simulink model "ds1_plant"  (R2019a)
settings: Solver=ode14x  StartTime=0  StopTime=0.166  FixedStep=.00001  RelTol=1e-3  EnableMultiTasking=on
model workspace (MAT data in the model file):
  Ankle_L_D = 0.125126243033
  Ankle_L_S = 0.0328154604487
  Ankle_R_D = 0.245807097642
  Ankle_R_S = 0.0328154604487
  BeginTimePlantModel = 0.1577
  F_C = 0.0618
  F_H = 0.107
  F_I = 0.0129
  F_L = 0.2471
  F_M = 1.2499
  F_W = 0.11
  GRF_HD = 941.037069119
  GRF_HS = 1691.11560066
  GRF_VD = 12300.8672242
  GRF_VS = 76710.3574634
  HAT_I = 4.3688
  HAT_L = 0.549
  HAT_M = 58.9152
  HAT_a = 0.2
  HAT_b = 0.13
  Hip_L_D = 0.0332143791481
  Hip_L_S = 0.0516603438036
  Hip_R_D = 0.145088103411
  Hip_R_S = 0.15911410017
  Knee_L_D = 0.0558982452805
  Knee_L_S = 0.00250387295429
  Knee_R_D = 0.0619293882143
  Knee_R_S = 0.0623339259595
  M : struct (value not decoded)
  S_I = 0.073
  S_L = 0.447
  S_M = 4.0083
  S_R1 = 0.06
  S_R2 = 0.08
  T_I = 0.2042
  T_L = 0.476
  T_M = 8.6199999
  T_R1 = 0.08
  T_R2 = 0.1
  bodymass = 2.85423037717
  p_stance_ankle = 14.9539905036
  p_stance_hip = -24.9413676415
  p_stance_knee = -2.50807459996
  p_swing_ankle = 4.11757124464
  p_swing_hip = 18.3000604838
  p_swing_knee = -3.41741510381
  polyfit_stance_ankle = [-863347.977095 222377.922877 -7468.35453889 -9.40558010807 -153.06789694]
  polyfit_stance_hip = [-279786636.688 114363391.625 -15725654.0525 856134.662579 -22930.0516399 481.110496147 63.2694363354]
  polyfit_stance_knee = [-122862314.114 52903969.6705 -7988612.27678 487806.049871 -8969.32141641 330.337585729 -54.0526736443]
  polyfit_swing_ankle = [49510154320.8 -30205907167.6 7312588550.85 -888915044.437 56385922.5861 -1769074.37171 25613.4020917 -113.306543933 -1.03720591697]
  polyfit_swing_hip = [538683495113 -366532634246 101719653645 -14750073882.9 1184454520.37 -50949861.1242 1019832.60417 -6310.84925925 -38.0907282261]
  polyfit_swing_knee = [352478408737 -233011269241 62650744932.5 -8775138187.04 678489689.503 -28060179.8998 545151.783137 -3282.03325692 -26.455631467]
  stance_hip_D = -0.1
  stance_hip_I = 0
  stance_hip_P = -1
  swing_hip_D = -0.1
  swing_hip_I = 0
  swing_hip_P = -1
  u_stance_ankle = [-114.620040933 -149.993105962 -149.909908907 -149.999889888 -149.999957965 -149.999973006]
  u_stance_knee = [-4.39803453247 -27.0219790006 -26.9634089217 -27.1316089475 -27.1524298795 -13.1129133696]
  u_swing_ankle = [7.00267747461 -1.55234842214 7.02970023555 7.00586724227 7.06043061801 0.00199706532211]
  u_swing_knee = [-10.6470024823 -8.89238612545 -13.3071794193 -13.064145722 -14.1272814659 -14.0994649135]
  w_stance_ankle = -19.9817779
  w_stance_hip = 18.2437977096
  w_stance_knee = 116.890654217
  w_swing_ankle = -56.5478745686
  w_swing_hip = 29.8978013919
  w_swing_knee = 6.91676966665
  x_planar_p = 0
  x_planar_v = 0
  y_planar_p = 0
  y_planar_v = 0
  yout = [8.16988597066 8.1627557225 8.15559878707 8.14841513681 8.14120474348 8.13396757813 8.12670361115 8.11941281227 8.1120951506 8.10475059463 8.09737911226 8.08998067083 ... (8000 elements, 1000x8)]
  z_planar_p = -10.3139246991
  z_planar_w = -47.4942945829
symbols that are objects in the model workspace (value not decoded): M
undefined symbols (not defined in the file or in its folder): X, Y, Z
libraries: nesl_utility x88, sm_lib x51, fl_lib x24, fl_ps_legacy_lib x16, simulink x4
(part 3 of 4)

== system ds1_plant/lead shank ==
  Rigid  Transform : sm_lib/Frames and Transforms/Rigid Transform  TranslationMethod=None  TranslationStandardOffset=S_L  TranslationLengthUnit=m  TranslationStandardAxis=+Z  TranslationCartesianOffset=[0 0 0]  TranslationROffset=0  TranslationROffsetUnits=m  TranslationZOffset=0  TranslationZOffsetUnits=m  TranslationThetaOffset=0  TranslationThetaOffsetUnits=deg  RotationMethod=StandardAxis  RotationAngleUnits=deg  RotationStandardAxis=+Y  RotationAngle=90  RotationArbitraryAxis=[0 0 1]  FollAlignAxisA=+X  BaseAlignAxisA=+Y  FollAlignAxisB=+Y  BaseAlignAxisB=+Z  RotationSequenceAxes=FollowerAxes  RotationSequence=XYX  RotationSequenceAngles=[0 0 0]  RotationSequenceAnglesUnits=deg  RotationMatrix=[1 0 0; 0 1 0; 0 0 1]
  Rigid  Transform1 : sm_lib/Frames and Transforms/Rigid Transform  TranslationMethod=StandardAxis  TranslationStandardOffset=S_L  TranslationLengthUnit=m  TranslationStandardAxis=+Z  TranslationCartesianOffset=[0 0 0]  TranslationROffset=0  TranslationROffsetUnits=m  TranslationZOffset=0  TranslationZOffsetUnits=m  TranslationThetaOffset=0  TranslationThetaOffsetUnits=deg  RotationMethod=StandardAxis  RotationAngleUnits=deg  RotationStandardAxis=+Y  RotationAngle=90  RotationArbitraryAxis=[0 0 1]  FollAlignAxisA=+X  BaseAlignAxisA=+Y  FollAlignAxisB=+Y  BaseAlignAxisB=+Z  RotationSequenceAxes=FollowerAxes  RotationSequence=XYX  RotationSequenceAngles=[0 0 0]  RotationSequenceAnglesUnits=deg  RotationMatrix=[1 0 0; 0 1 0; 0 0 1]
  Solid : sm_lib/Body Elements/Solid  InertiaType=Custom  Mass=S_M  MassUnits=kg  CenterOfMass=[0 0 0.567*S_L]  CenterOfMassUnits=m  MomentsOfInertia=[S_I .001 .001]  MomentsOfInertiaUnits=kg*m^2  ProductsOfInertia=[0 0 0]  ProductsOfInertiaUnits=kg*m^2  BasedOnType=Density  Density=0  DensityUnits=kg/(m^3)  DoExposeReferenceFrame=on  SerializedFrames=<Frames/>  GraphicType=FromGeometry  MarkerShape=Sphere  MarkerSize=10  MarkerSizeUnits=m  GraphicVisPropType=SimpleVisualProperties  GraphicDiffuseColor=[0.0 0.4 1.0]  GraphicSpecularColor=[0.5 0.5 0.5 1.0]  GraphicAmbientColor=[0.15 0.15 0.15 1.0]  GraphicEmissiveColor=[0.0 0.0 0.0 1.0]  GraphicShininess=75  GraphicOpacity=1.0  GeometryShape=GeneralSolidOfRevolution  RectangleSize=[1 1]  RectangleSizeUnits=m  BrickDimensions=[1 1 1]  BrickDimensionUnits=m  CylinderRadius=1  CylinderRadiusUnits=m  CylinderLength=1  CylinderLengthUnits=m  SphereRadius=1  SphereRadiusUnits=m  EllipsoidRadii=[1 1 1]  EllipsoidRadiiUnits=m  ExtrusionCrossSection=[1 1; -1 1; -1 -1; 1 -1]  ExtrusionCrossSectionUnits=m  ExtrusionLength=1  ExtrusionLengthUnits=m  PolygonNumSides=3  PolygonOuterRadius=1  PolygonOuterRadiusUnits=m  ExtGeomFileType=STEP  ExtGeomFileUnits=m  RevolutionCrossSection=S_cross_section  RevolutionCrossSectionUnits=m  RevolutionExtent=Full  RevolutionAngle=180  RevolutionAngleUnits=deg
  B : PMIOPort  Side=Right
  F : PMIOPort  Port=2  Side=Left
  connections:
  B/RConn1 -- Rigid  Transform/RConn1
  Rigid  Transform/LConn1 -- Rigid  Transform1/LConn1 -- Solid/RConn1
  F/RConn1 -- Rigid  Transform1/RConn1

== system ds1_plant/lead thigh ==
  Rigid  Transform : sm_lib/Frames and Transforms/Rigid Transform  TranslationMethod=None  TranslationStandardOffset=T_L  TranslationLengthUnit=m  TranslationStandardAxis=+Z  TranslationCartesianOffset=[0 0 0]  TranslationROffset=0  TranslationROffsetUnits=m  TranslationZOffset=0  TranslationZOffsetUnits=m  TranslationThetaOffset=0  TranslationThetaOffsetUnits=deg  RotationMethod=StandardAxis  RotationAngleUnits=deg  RotationStandardAxis=+Y  RotationAngle=90  RotationArbitraryAxis=[0 0 1]  FollAlignAxisA=+X  BaseAlignAxisA=+Y  FollAlignAxisB=+Y  BaseAlignAxisB=+Z  RotationSequenceAxes=FollowerAxes  RotationSequence=XYX  RotationSequenceAngles=[0 0 0]  RotationSequenceAnglesUnits=deg  RotationMatrix=[1 0 0; 0 1 0; 0 0 1]
  Rigid  Transform1 : sm_lib/Frames and Transforms/Rigid Transform  TranslationMethod=StandardAxis  TranslationStandardOffset=T_L  TranslationLengthUnit=m  TranslationStandardAxis=+Z  TranslationCartesianOffset=[0 0 0]  TranslationROffset=0  TranslationROffsetUnits=m  TranslationZOffset=0  TranslationZOffsetUnits=m  TranslationThetaOffset=0  TranslationThetaOffsetUnits=deg  RotationMethod=StandardAxis  RotationAngleUnits=deg  RotationStandardAxis=+Y  RotationAngle=90  RotationArbitraryAxis=[0 0 1]  FollAlignAxisA=+X  BaseAlignAxisA=+Y  FollAlignAxisB=+Y  BaseAlignAxisB=+Z  RotationSequenceAxes=FollowerAxes  RotationSequence=XYX  RotationSequenceAngles=[0 0 0]  RotationSequenceAnglesUnits=deg  RotationMatrix=[1 0 0; 0 1 0; 0 0 1]
  Thigh : sm_lib/Body Elements/Solid  InertiaType=Custom  Mass=T_M  MassUnits=kg  CenterOfMass=[0 0 0.567*T_L]  CenterOfMassUnits=m  MomentsOfInertia=[T_I .001 .001]  MomentsOfInertiaUnits=kg*m^2  ProductsOfInertia=[0 0 0]  ProductsOfInertiaUnits=kg*m^2  BasedOnType=Density  Density=0  DensityUnits=kg/(m^3)  DoExposeReferenceFrame=on  SerializedFrames=<Frames/>  GraphicType=FromGeometry  MarkerShape=Sphere  MarkerSize=10  MarkerSizeUnits=m  GraphicVisPropType=SimpleVisualProperties  GraphicDiffuseColor=[0.0 0.4 1.0]  GraphicSpecularColor=[0.5 0.5 0.5 1.0]  GraphicAmbientColor=[0.15 0.15 0.15 1.0]  GraphicEmissiveColor=[0.0 0.0 0.0 1.0]  GraphicShininess=75  GraphicOpacity=1.0  GeometryShape=GeneralSolidOfRevolution  RectangleSize=[1 1]  RectangleSizeUnits=m  BrickDimensions=[1 1 1]  BrickDimensionUnits=m  CylinderRadius=[1 2]  CylinderRadiusUnits=m  CylinderLength=1  CylinderLengthUnits=m  SphereRadius=1  SphereRadiusUnits=m  EllipsoidRadii=[1 1 1]  EllipsoidRadiiUnits=m  ExtrusionCrossSection=T_cross_section  ExtrusionCrossSectionUnits=cm  ExtrusionLength=T_L  ExtrusionLengthUnits=cm  PolygonNumSides=3  PolygonOuterRadius=1  PolygonOuterRadiusUnits=m  ExtGeomFileType=STEP  ExtGeomFileUnits=m  RevolutionCrossSection=T_cross_section  RevolutionCrossSectionUnits=m  RevolutionExtent=Full  RevolutionAngle=180  RevolutionAngleUnits=deg
  B : PMIOPort  Side=Right
  F : PMIOPort  Port=2  Side=Left
  connections:
  B/RConn1 -- Rigid  Transform/RConn1
  Rigid  Transform/LConn1 -- Rigid  Transform1/LConn1 -- Thigh/RConn1
  Rigid  Transform1/RConn1 -- F/RConn1

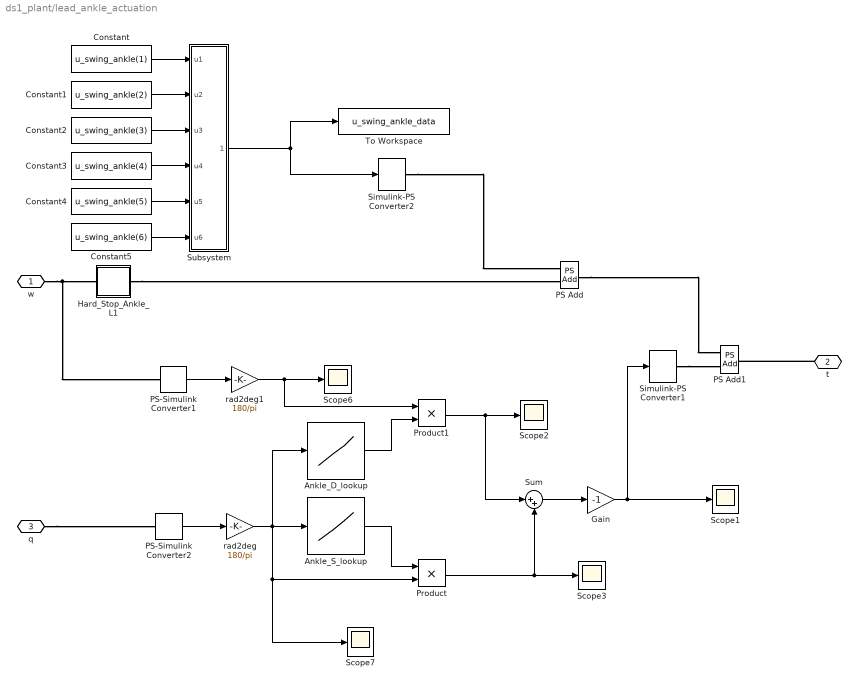
== system ds1_plant/lead_ankle_actuation ==
  Ankle_D_lookup : Lookup_n-D  NumberOfTableDimensions=1  BreakpointsForDimension1=[-45:.01:20]  Table=[exp(linspace(log(1000),log(.01),1000)), zeros(1,4500),exp(linspace(log(.01),log(1000),1001))]  RndMeth=Simplest  InputSameDT=on
  Ankle_S_lookup : Lookup_n-D  NumberOfTableDimensions=1  BreakpointsForDimension1=[-45:.01:20]  Table=[exp(linspace(log(10000),log(.01),1000)), zeros(1,4500),exp(linspace(log(.01),log(10000),1001))]  RndMeth=Simplest  InputSameDT=on
  Constant : Constant  Value=u_swing_ankle(1)
  Constant1 : Constant  Value=u_swing_ankle(2)
  Constant2 : Constant  Value=u_swing_ankle(3)
  Constant3 : Constant  Value=u_swing_ankle(4)
  Constant4 : Constant  Value=u_swing_ankle(5)
  Constant5 : Constant  Value=u_swing_ankle(6)
  Gain : Gain  Gain=-1
  Hard_Stop_Ankle_L1 : Subsystem  mask{upper_bound=((20-p_swing_ankle)*pi)/180, lower_bound=((-45-p_swing_ankle)*pi)/180, contact_stiffness=1e8, contact_damping=5000, initial_angular_position=0}
      mask prompts: upper_bound "Upper Bound"; lower_bound "Lower Bound"; contact_stiffness "Contact Stiffness"; contact_damping "Contact Damping"; initial_angular_position "Initial Angular Position"
  PS Add : fl_ps_legacy_lib/Legacy Physical Signals/Functions/PS Add
      settings: SourceProductName=Simscape  SourceProductBaseCode=SS
  PS Add1 : fl_ps_legacy_lib/Legacy Physical Signals/Functions/PS Add
      settings: SourceProductName=Simscape  SourceProductBaseCode=SS
  PS-Simulink Converter1 : nesl_utility/PS-Simulink Converter  PhysicalDomain=network_engine_domain  SubClassName=ps_output  LeftPortType=input  RightPortType=output  PseudoPeriodic=off  Frequencies=[]  Unit=1  AffineConversion=off
  PS-Simulink Converter2 : nesl_utility/PS-Simulink Converter  PhysicalDomain=network_engine_domain  SubClassName=ps_output  LeftPortType=input  RightPortType=output  PseudoPeriodic=off  Frequencies=[]  Unit=1  AffineConversion=off
  Product : Product  RndMeth=Zero
  Product1 : Product  RndMeth=Zero
  Scope{1..3,6..7} (5 alike) : Scope
  Simulink-PS Converter1 : nesl_utility/Simulink-PS Converter  PhysicalDomain=network_engine_domain  SubClassName=ps_input  LeftPortType=input  RightPortType=output  PseudoPeriodic=off  Frequencies=[]  NoiseDistribution=none  NoiseParameters=[]  Unit=1  AffineConversion=off  FilteringAndDerivatives=zero  SimscapeFilterOrder=1  InputFilterTimeConstant=.001  UdotUserProvided=[]
  Simulink-PS Converter2 : nesl_utility/Simulink-PS Converter  PhysicalDomain=network_engine_domain  SubClassName=ps_input  LeftPortType=input  RightPortType=output  PseudoPeriodic=off  Frequencies=[]  NoiseDistribution=none  NoiseParameters=[]  Unit=1  AffineConversion=off  FilteringAndDerivatives=zero  SimscapeFilterOrder=1  InputFilterTimeConstant=.001  UdotUserProvided=[]
  Subsystem : Subsystem
  Sum : Sum  Inputs=|++
  To Workspace : ToWorkspace  VariableName=u_swing_ankle_data  SampleTime=-1
  rad2deg : Gain  Gain=180/pi
  "rad2deg1 " : Gain  Gain=180/pi
  w : PMIOPort  Side=Right
  t : PMIOPort  Port=2  Side=Left
  q : PMIOPort  Port=3  Side=Right
  wires:
  PS-Simulink Converter1/1 -> "rad2deg1 "/1
  PS-Simulink Converter2/1 -> rad2deg/1
  rad2deg/1 -> Ankle_D_lookup/1, Scope7/1, Product/2, Ankle_S_lookup/1
  Ankle_S_lookup/1 -> Product/1
  "rad2deg1 "/1 -> Product1/1, Scope6/1
  Product1/1 -> Sum/1, Scope2/1
  Product/1 -> Scope3/1, Sum/2
  Sum/1 -> Gain/1
  Gain/1 -> Simulink-PS Converter1/1, Scope1/1
  Ankle_D_lookup/1 -> Product1/2
  Constant/1 -> Subsystem/1(u1)
  Constant1/1 -> Subsystem/2(u2)
  Constant2/1 -> Subsystem/3(u3)
  Constant3/1 -> Subsystem/4(u4)
  Constant4/1 -> Subsystem/5(u5)
  Subsystem/1(Out1) -> To Workspace/1, Simulink-PS Converter2/1
  Constant5/1 -> Subsystem/6(u6)
  connections:
  w/RConn1 -- PS-Simulink Converter1/LConn1 -- Hard_Stop_Ankle_L1/LConn1
  Hard_Stop_Ankle_L1/RConn1 -- PS Add/LConn2
  t/RConn1 -- PS Add1/RConn1
  q/RConn1 -- PS-Simulink Converter2/LConn1
  PS Add/RConn1 -- PS Add1/LConn1
  Simulink-PS Converter1/RConn1 -- PS Add1/LConn2
  Simulink-PS Converter2/RConn1 -- PS Add/LConn1

== system ds1_plant/lead_hip_actuation ==
  HAT_feedback : Inport
  HAT_reference : Constant  Value=0
  Hip_R_Actuation1 : Subsystem
  Scope : Scope
  Sum : Sum  Inputs=|+-
  Swing_hip_PID : Subsystem
  q : PMIOPort  Side=Right
  t : PMIOPort  Port=2  Side=Left
  w : PMIOPort  Port=3  Side=Right
  wires:
  HAT_feedback/1 -> Sum/2
  Sum/1 -> Swing_hip_PID/1(Error)
  HAT_reference/1 -> Sum/1
  Swing_hip_PID/1(Swing_hip_control_moment) -> Scope/1, Hip_R_Actuation1/1(Swing_hip_moment)
  connections:
  q/RConn1 -- Hip_R_Actuation1/RConn2
  t/RConn1 -- Hip_R_Actuation1/LConn1
  w/RConn1 -- Hip_R_Actuation1/RConn1

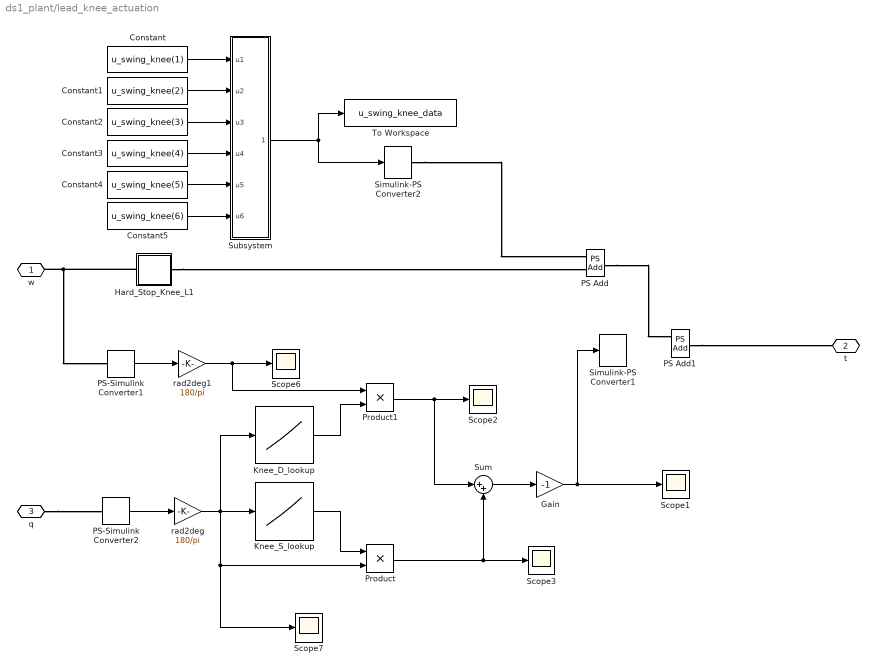
== system ds1_plant/lead_knee_actuation ==
  Constant : Constant  Value=u_swing_knee(1)
  Constant1 : Constant  Value=u_swing_knee(2)
  Constant2 : Constant  Value=u_swing_knee(3)
  Constant3 : Constant  Value=u_swing_knee(4)
  Constant4 : Constant  Value=u_swing_knee(5)
  Constant5 : Constant  Value=u_swing_knee(6)
  Gain : Gain  Gain=-1
  Hard_Stop_Knee_L1 : Subsystem  mask{upper_bound=(-p_swing_knee*pi)/180, lower_bound=((-140-p_swing_knee)*pi)/180, contact_stiffness=1e8, contact_damping=5000, initial_angular_position=0}
      mask prompts: upper_bound "Upper Bound"; lower_bound "Lower Bound"; contact_stiffness "Contact Stiffness"; contact_damping "Contact Damping"; initial_angular_position "Initial Angular Position"
  Knee_D_lookup : Lookup_n-D  NumberOfTableDimensions=1  BreakpointsForDimension1=[-140:.01:0]  Table=[exp(linspace(log(1000),log(.01),1000)), zeros(1,12000),exp(linspace(log(.01),log(1000),1001))]  RndMeth=Simplest  InputSameDT=on
  Knee_S_lookup : Lookup_n-D  NumberOfTableDimensions=1  BreakpointsForDimension1=[-140:.01:0]  Table=[exp(linspace(log(10000),log(.01),1000)), zeros(1,12000),exp(linspace(log(.01),log(10000),1001))]  RndMeth=Simplest  InputSameDT=on
  PS Add : fl_ps_legacy_lib/Legacy Physical Signals/Functions/PS Add
      settings: SourceProductName=Simscape  SourceProductBaseCode=SS
  PS Add1 : fl_ps_legacy_lib/Legacy Physical Signals/Functions/PS Add
      settings: SourceProductName=Simscape  SourceProductBaseCode=SS
  PS-Simulink Converter1 : nesl_utility/PS-Simulink Converter  PhysicalDomain=network_engine_domain  SubClassName=ps_output  LeftPortType=input  RightPortType=output  PseudoPeriodic=off  Frequencies=[]  Unit=1  AffineConversion=off
  PS-Simulink Converter2 : nesl_utility/PS-Simulink Converter  PhysicalDomain=network_engine_domain  SubClassName=ps_output  LeftPortType=input  RightPortType=output  PseudoPeriodic=off  Frequencies=[]  Unit=1  AffineConversion=off
  Product : Product  RndMeth=Zero
  Product1 : Product  RndMeth=Zero
  Scope{1..3,6..7} (5 alike) : Scope
  Simulink-PS Converter1 : nesl_utility/Simulink-PS Converter  PhysicalDomain=network_engine_domain  SubClassName=ps_input  LeftPortType=input  RightPortType=output  PseudoPeriodic=off  Frequencies=[]  NoiseDistribution=none  NoiseParameters=[]  Unit=1  AffineConversion=off  FilteringAndDerivatives=zero  SimscapeFilterOrder=1  InputFilterTimeConstant=.001  UdotUserProvided=[]
  Simulink-PS Converter2 : nesl_utility/Simulink-PS Converter  PhysicalDomain=network_engine_domain  SubClassName=ps_input  LeftPortType=input  RightPortType=output  PseudoPeriodic=off  Frequencies=[]  NoiseDistribution=none  NoiseParameters=[]  Unit=1  AffineConversion=off  FilteringAndDerivatives=zero  SimscapeFilterOrder=1  InputFilterTimeConstant=.001  UdotUserProvided=[]
  Subsystem : Subsystem
  Sum : Sum  Inputs=|++
  To Workspace : ToWorkspace  VariableName=u_swing_knee_data  SampleTime=-1
  rad2deg : Gain  Gain=180/pi
  "rad2deg1 " : Gain  Gain=180/pi
  w : PMIOPort  Side=Right
  t : PMIOPort  Port=2  Side=Left
  q : PMIOPort  Port=3  Side=Right
  wires:
  PS-Simulink Converter1/1 -> "rad2deg1 "/1
  PS-Simulink Converter2/1 -> rad2deg/1
  rad2deg/1 -> Knee_S_lookup/1, Knee_D_lookup/1, Scope7/1, Product/2
  Knee_S_lookup/1 -> Product/1
  "rad2deg1 "/1 -> Product1/1, Scope6/1
  Product1/1 -> Sum/1, Scope2/1
  Product/1 -> Scope3/1, Sum/2
  Sum/1 -> Gain/1
  Gain/1 -> Simulink-PS Converter1/1, Scope1/1
  Knee_D_lookup/1 -> Product1/2
  Constant/1 -> Subsystem/1(u1)
  Constant1/1 -> Subsystem/2(u2)
  Constant2/1 -> Subsystem/3(u3)
  Constant3/1 -> Subsystem/4(u4)
  Constant4/1 -> Subsystem/5(u5)
  Subsystem/1(Out1) -> Simulink-PS Converter2/1, To Workspace/1
  Constant5/1 -> Subsystem/6(u6)
  connections:
  Hard_Stop_Knee_L1/LConn1 -- PS-Simulink Converter1/LConn1 -- w/RConn1
  q/RConn1 -- PS-Simulink Converter2/LConn1
  PS Add/RConn1 -- PS Add1/LConn1
  PS Add1/RConn1 -- t/RConn1
  Hard_Stop_Knee_L1/RConn1 -- PS Add/LConn2
  Simulink-PS Converter2/RConn1 -- PS Add/LConn1

== system ds1_plant/HAT/vCOMCal1 ==
  PS-S : nesl_utility/PS-Simulink Converter  PhysicalDomain=network_engine_domain  SubClassName=ps_output  LeftPortType=input  RightPortType=output  PseudoPeriodic=off  Frequencies=[]  Unit=1  AffineConversion=off
  PS-S1 : nesl_utility/PS-Simulink Converter  PhysicalDomain=network_engine_domain  SubClassName=ps_output  LeftPortType=input  RightPortType=output  PseudoPeriodic=off  Frequencies=[]  Unit=1  AffineConversion=off
  Transform Sensor : sm_lib/Frames and Transforms/Transform Sensor  MeasurementFrame=World  SenseAngle=off  SenseAxis=off  SenseAngle1=off  SenseAngle2=off  SenseAngle3=off  SenseQ=off  SenseR=off  SenseOmegaX=off  SenseOmegaY=off  SenseOmegaZ=off  SenseOmega1=off  SenseOmega2=off  SenseOmega3=off  SenseQDot=off  SenseRDot=off  SenseAlphaX=off  SenseAlphaY=off  SenseAlphaZ=off  SenseAlpha1=off  SenseAlpha2=off  SenseAlpha3=off  SenseQDDot=off  SenseRDDot=off  SenseX=off  SenseY=off  SenseZ=off  SenseRad=off  SenseAzim=off  SenseDist=off  SenseInc=off  SenseXDot=off  SenseYDot=on  SenseZDot=on  SenseRadDot=off  SenseAzimDot=off  SenseDistDot=off  SenseIncDot=off  SenseXDDot=off  SenseYDDot=off  SenseZDDot=off  SenseRadDDot=off  SenseAzimDDot=off  SenseDistDDot=off  SenseIncDDot=off
  Conn2 : PMIOPort  Side=Left
  vCOM_y : Outport
  vCOM_z : Outport  Port=2
  wires:
  PS-S/1 -> vCOM_y/1
  PS-S1/1 -> vCOM_z/1
  connections:
  Transform Sensor/RConn2 -- PS-S/LConn1
  Transform Sensor/RConn1 -- Conn2/RConn1
  Transform Sensor/RConn3 -- PS-S1/LConn1

== system ds1_plant/lag foot/Heel_GRF ==
  External Force  and Torque : sm_lib/Forces and Torques/External Force and Torque  ForceResolutionFrame=World  EnableForceX=off  EnableForceY=on  EnableForceZ=on  EnableForce=off  TorqueResolutionFrame=AttachedFrame  EnableTorqueX=off  EnableTorqueY=off  EnableTorqueZ=off  EnableTorque=off
  Heel Sensor : sm_lib/Frames and Transforms/Transform Sensor  MeasurementFrame=World  SenseAngle=off  SenseAxis=off  SenseAngle1=off  SenseAngle2=off  SenseAngle3=off  SenseQ=off  SenseR=off  SenseOmegaX=off  SenseOmegaY=off  SenseOmegaZ=off  SenseOmega1=off  SenseOmega2=off  SenseOmega3=off  SenseQDot=off  SenseRDot=off  SenseAlphaX=off  SenseAlphaY=off  SenseAlphaZ=off  SenseAlpha1=off  SenseAlpha2=off  SenseAlpha3=off  SenseQDDot=off  SenseRDDot=off  SenseX=off  SenseY=on  SenseZ=on  SenseRad=off  SenseAzim=off  SenseDist=off  SenseInc=off  SenseXDot=off  SenseYDot=on  SenseZDot=on  SenseRadDot=off  SenseAzimDot=off  SenseDistDot=off  SenseIncDot=off  SenseXDDot=off  SenseYDDot=off  SenseZDDot=off  SenseRadDDot=off  SenseAzimDDot=off  SenseDistDDot=off  SenseIncDDot=off
  Subsystem : Subsystem
  Subsystem1 : Subsystem
  Heel : PMIOPort  Side=Left
  connections:
  Subsystem1/RConn1 -- External Force  and Torque/LConn1
  Heel Sensor/RConn4 -- Subsystem1/LConn3
  Heel Sensor/RConn2 -- Subsystem1/LConn2
  Heel Sensor/RConn5 -- Subsystem/LConn2
  Heel/RConn1 -- Heel Sensor/RConn1 -- External Force  and Torque/RConn1
  Subsystem/LConn1 -- Subsystem1/LConn1 -- Heel Sensor/RConn3
  Subsystem/RConn1 -- External Force  and Torque/LConn2

== system ds1_plant/lag foot/Toe_GRF ==
  External Force  and Torque : sm_lib/Forces and Torques/External Force and Torque  ForceResolutionFrame=World  EnableForceX=off  EnableForceY=on  EnableForceZ=on  EnableForce=off  TorqueResolutionFrame=AttachedFrame  EnableTorqueX=off  EnableTorqueY=off  EnableTorqueZ=off  EnableTorque=off
  Heel Sensor : sm_lib/Frames and Transforms/Transform Sensor  MeasurementFrame=World  SenseAngle=off  SenseAxis=off  SenseAngle1=off  SenseAngle2=off  SenseAngle3=off  SenseQ=off  SenseR=off  SenseOmegaX=off  SenseOmegaY=off  SenseOmegaZ=off  SenseOmega1=off  SenseOmega2=off  SenseOmega3=off  SenseQDot=off  SenseRDot=off  SenseAlphaX=off  SenseAlphaY=off  SenseAlphaZ=off  SenseAlpha1=off  SenseAlpha2=off  SenseAlpha3=off  SenseQDDot=off  SenseRDDot=off  SenseX=off  SenseY=on  SenseZ=on  SenseRad=off  SenseAzim=off  SenseDist=off  SenseInc=off  SenseXDot=off  SenseYDot=on  SenseZDot=on  SenseRadDot=off  SenseAzimDot=off  SenseDistDot=off  SenseIncDot=off  SenseXDDot=off  SenseYDDot=off  SenseZDDot=off  SenseRadDDot=off  SenseAzimDDot=off  SenseDistDDot=off  SenseIncDDot=off
  Subsystem : Subsystem
  Subsystem1 : Subsystem
  Toe : PMIOPort  Side=Left
  lag toe grf z : Outport
  wires:
  Subsystem/1(lag toe grf z) -> lag toe grf z/1
  connections:
  Subsystem1/RConn1 -- External Force  and Torque/LConn1
  Heel Sensor/RConn4 -- Subsystem1/LConn3
  Heel Sensor/RConn2 -- Subsystem1/LConn2
  Heel Sensor/RConn5 -- Subsystem/LConn2
  Heel Sensor/RConn1 -- Toe/RConn1 -- External Force  and Torque/RConn1
  Subsystem1/LConn1 -- Heel Sensor/RConn3 -- Subsystem/LConn1
  Subsystem/RConn1 -- External Force  and Torque/LConn2

== system ds1_plant/lag_ankle_actuation/Hard_Stop_Ankle_L ==
  Mechanical Rotational Reference : fl_lib/Mechanical/Rotational Elements/Mechanical Rotational Reference
  Rotational Simscape Intf (Library Block) : Subsystem
  Rotational Hard Stop : fl_lib/Mechanical/Rotational Elements/Rotational Hard Stop  upper_bnd=upper_bound rad  lower_bnd=lower_bound rad  stiff_up=contact_stiffness N*m/rad  stiff_low=contact_stiffness N*m/rad  D_up=contact_damping N*m/(rad/s)  D_low=contact_damping N*m/(rad/s)  model=3  transition=0.001 rad  w_specify=off  w_priority=None  w=0 rad/s  w_nominal_specify=off  w_nominal_unit=rad/s  w_nominal_value=1  t_specify=off  t_priority=None  t=0 N*m  t_nominal_specify=off  t_nominal_unit=N*m  t_nominal_value=1  phi_specify=on  phi_priority=High  phi=initial_angular_position rad  phi_nominal_specify=off  phi_nominal_unit=rad  phi_nominal_value=1
      settings: SourceProductName=Simscape  SourceProductBaseCode=SS
  T : PMIOPort  Side=Right
  w : PMIOPort  Port=2  Side=Left
  connections:
  Rotational Simscape Intf (Library Block)/LConn2 -- Rotational Hard Stop/LConn1 -- Mechanical Rotational Reference/LConn1
  Rotational Hard Stop/RConn1 -- Rotational Simscape Intf (Library Block)/RConn2
  w/RConn1 -- Rotational Simscape Intf (Library Block)/LConn1
  Rotational Simscape Intf (Library Block)/RConn1 -- T/RConn1

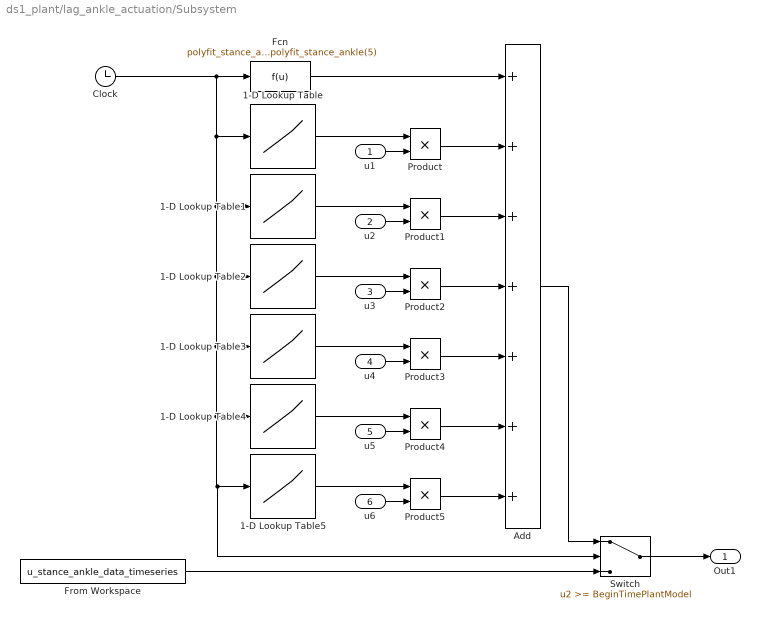
== system ds1_plant/lag_ankle_actuation/Subsystem ==
  u1 : Inport
  u2 : Inport  Port=2
  u3 : Inport  Port=3
  u4 : Inport  Port=4
  u5 : Inport  Port=5
  u6 : Inport  Port=6
  1-D Lookup Table : Lookup_n-D  NumberOfTableDimensions=1  BreakpointsForDimension1=0:0.166/20:0.166  Table="[0.828492607088319\t0.463955859969459\t0.259815281582897\t0.145496557686422\t0.0814780723043965\t0.0456277204904620\t0.0255515234746587\t0.0143088531458089\t0.00801295776165298\t0.00448725634652567\t0.00251286355405438\t0.00140720359027045\t0.000788034010551453\t0.000441299045908813\t0.000247127465708936\t0.000138391380797004\t7.74991732463222e-05\t4.33995370179404e-05\t2.43037407300467e-05\t1.36100948088261e-05\t7.62165309294263e-06]"  InternalRulePriority=Speed  RndMeth=Simplest  InputSameDT=on
  1-D Lookup Table1 : Lookup_n-D  NumberOfTableDimensions=1  BreakpointsForDimension1=0:0.166/20:0.166  Table="[-0.463955859969459\t0.308862043922525\t0.491422046879651\t0.453533555531105\t0.353847628293379\t0.254081220674030\t0.173604350922110\t0.114757002229387\t0.0740855180477401\t0.0469879843143331\t0.0293933239722817\t0.0181850909679807\t0.0111495554864308\t0.00678465761724378\t0.00410231593076833\t0.00246692521369288\t0.00147646996344708\t0.000880018612046638\t0.000522599864955231\t0.000309338012012034\t0.000182571255803517]"  InternalRulePriority=Speed  RndMeth=Simplest  InputSameDT=on
  1-D Lookup Table2 : Lookup_n-D  NumberOfTableDimensions=1  BreakpointsForDimension1=0:0.166/20:0.166  Table="[0.259815281582897\t-0.491422046879651\t-0.241530648582683\t0.102186092575929\t0.312603095529333\t0.386619878212349\t0.373369915956564\t0.318427582609329\t0.251588558383877\t0.188661839526685\t0.136178353024799\t0.0954695507240998\t0.0654042883010754\t0.0439765486693765\t0.0291142279508644\t0.0190248054635844\t0.0122939930937698\t0.00786829567321203\t0.00499360826467044\t0.00314579120644394\t0.00196874118437067]"  InternalRulePriority=Speed  RndMeth=Simplest  InputSameDT=on
  1-D Lookup Table3 : Lookup_n-D  NumberOfTableDimensions=1  BreakpointsForDimension1=0:0.166/20:0.166  Table="[-0.145496557686422\t0.453533555531105\t-0.102186092575929\t-0.355979072267724\t-0.272219921390423\t-0.0563471922482192\t0.145978297617670\t0.276798316361235\t0.332545047076649\t0.332163154611857\t0.298413328415437\t0.249826868531948\t0.198746195653388\t0.152075290612122\t0.112834743759681\t0.0816477933966784\t0.0578629336332132\t0.0402909903513704\t0.0276348296417640\t0.0187074697884497\t0.0125194792247282]"  InternalRulePriority=Speed  RndMeth=Simplest  InputSameDT=on
  1-D Lookup Table4 : Lookup_n-D  NumberOfTableDimensions=1  BreakpointsForDimension1=0:0.166/20:0.166  Table="[0.0814780723043965\t-0.353847628293379\t0.312603095529333\t0.272219921390423\t-0.0510927603104505\t-0.269277439505272\t-0.288890405037067\t-0.170807386365379\t-0.00507904636630098\t0.143689414528881\t0.245517762835385\t0.296000229225362\t0.304289127332253\t0.283985944216662\t0.247919962868031\t0.205947158663638\t0.164574959413716\t0.127461956308127\t0.0961941812845337\t0.0710273880795710\t0.0514718987471617]"  InternalRulePriority=Speed  RndMeth=Simplest  InputSameDT=on
  1-D Lookup Table5 : Lookup_n-D  NumberOfTableDimensions=1  BreakpointsForDimension1=0:0.166/20:0.166  Table="[-0.0456277204904620\t0.254081220674030\t-0.386619878212348\t-0.0563471922482191\t0.269277439505272\t0.250497971935455\t0.0327800515993398\t-0.174881439776825\t-0.265896726675272\t-0.234447285440627\t-0.125091012505686\t0.00970666746599808\t0.131034051700259\t0.218636067523068\t0.267586962823482\t0.282438253197544\t0.271950603182582\t0.245488601663411\t0.211066831720298\t0.174616269723341\t0.139988235826231]"  InternalRulePriority=Speed  RndMeth=Simplest  InputSameDT=on
  Add : Sum  Inputs=+++++++
  Clock : Clock
  Fcn : Fcn  Expr=polyfit_stance_ankle(1)*u^4+polyfit_stance_ankle(2)*u^3+polyfit_stance_ankle(3)*u^2+polyfit_stance_ankle(4)*u+polyfit_stance_ankle(5)
  From Workspace : FromWorkspace  VariableName=u_stance_ankle_data_timeseries  SampleTime=0
  Product{,1..5} (6 alike) : Product
  Switch : Switch  Threshold=BeginTimePlantModel
  Out1 : Outport
  wires:
  Clock/1 -> 1-D Lookup Table/1, 1-D Lookup Table1/1, 1-D Lookup Table2/1, 1-D Lookup Table3/1, 1-D Lookup Table4/1, 1-D Lookup Table5/1, Switch/2, Fcn/1
  1-D Lookup Table/1 -> Product/1
  u1/1 -> Product/2
  1-D Lookup Table1/1 -> Product1/1
  u2/1 -> Product1/2
  1-D Lookup Table2/1 -> Product2/1
  u3/1 -> Product2/2
  1-D Lookup Table3/1 -> Product3/1
  u4/1 -> Product3/2
  1-D Lookup Table4/1 -> Product4/1
  u5/1 -> Product4/2
  1-D Lookup Table5/1 -> Product5/1
  u6/1 -> Product5/2
  Fcn/1 -> Add/1
  Product/1 -> Add/2
  Product1/1 -> Add/3
  Product2/1 -> Add/4
  Product3/1 -> Add/5
  Product4/1 -> Add/6
  Product5/1 -> Add/7
  Add/1 -> Switch/1
  From Workspace/1 -> Switch/3
  Switch/1 -> Out1/1

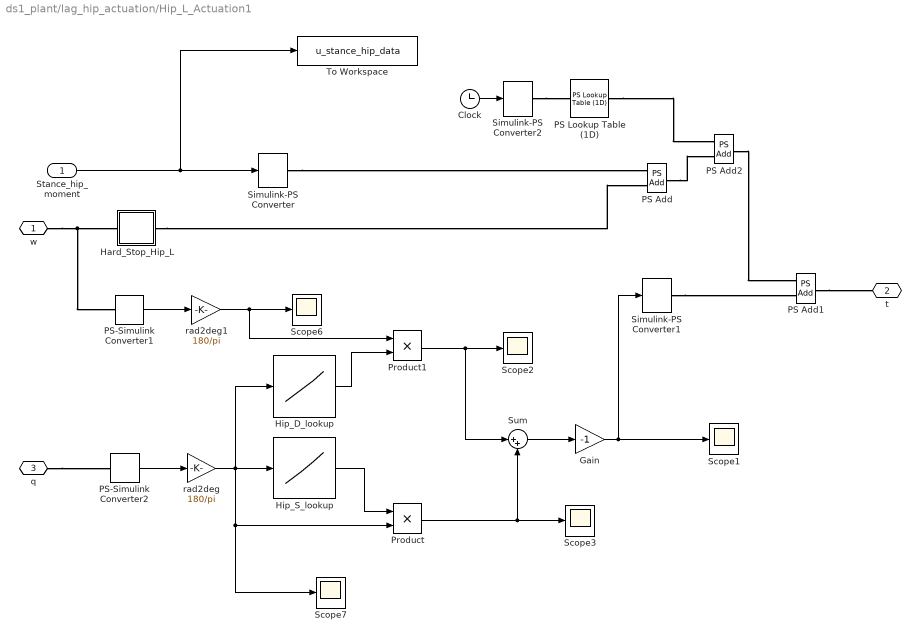
== system ds1_plant/lag_hip_actuation/Hip_L_Actuation1 ==
  Stance_hip_moment : Inport
  Clock : Clock
  Gain : Gain  Gain=-1
  Hard_Stop_Hip_L : Subsystem  mask{upper_bound=((125-p_stance_hip)*pi)/180, lower_bound=((-30-p_stance_hip)*pi)/180, contact_stiffness=1e8, contact_damping=5000, initial_angular_position=0}
      mask prompts: upper_bound "Upper Bound"; lower_bound "Lower Bound"; contact_stiffness "Contact Stiffness"; contact_damping "Contact Damping"; initial_angular_position "Initial Angular Position"
  Hip_D_lookup : Lookup_n-D  NumberOfTableDimensions=1  BreakpointsForDimension1=[-30:.01:125]  Table=[exp(linspace(log(1000),log(.01),1000)), zeros(1,13500),exp(linspace(log(.01),log(1000),1001))]  RndMeth=Simplest  InputSameDT=on
  Hip_S_lookup : Lookup_n-D  NumberOfTableDimensions=1  BreakpointsForDimension1=[-30:.01:125]  Table=[exp(linspace(log(10000),log(.01),1000)), zeros(1,13500),exp(linspace(log(.01),log(10000),1001))]  RndMeth=Simplest  InputSameDT=on
  PS Add : fl_ps_legacy_lib/Legacy Physical Signals/Functions/PS Add
      settings: SourceProductName=Simscape  SourceProductBaseCode=SS
  PS Add1 : fl_ps_legacy_lib/Legacy Physical Signals/Functions/PS Add
      settings: SourceProductName=Simscape  SourceProductBaseCode=SS
  PS Add2 : fl_ps_legacy_lib/Legacy Physical Signals/Functions/PS Add
      settings: SourceProductName=Simscape  SourceProductBaseCode=SS
  PS Lookup Table (1D) : fl_ps_legacy_lib/Legacy Physical Signals/Lookup Tables/PS Lookup Table (1D)  x=linspace(0,.1667,21)'  f=(-M.stance_hip/1000)*bodymass  interp_method=2  extrap_method=1
      settings: SourceProductName=Simscape  SourceProductBaseCode=SS
  PS-Simulink Converter1 : nesl_utility/PS-Simulink Converter  PhysicalDomain=network_engine_domain  SubClassName=ps_output  LeftPortType=input  RightPortType=output  PseudoPeriodic=off  Frequencies=[]  Unit=1  AffineConversion=off
  PS-Simulink Converter2 : nesl_utility/PS-Simulink Converter  PhysicalDomain=network_engine_domain  SubClassName=ps_output  LeftPortType=input  RightPortType=output  PseudoPeriodic=off  Frequencies=[]  Unit=1  AffineConversion=off
  Product : Product  RndMeth=Zero
  Product1 : Product  RndMeth=Zero
  Scope{1..3,6..7} (5 alike) : Scope
  Simulink-PS Converter : nesl_utility/Simulink-PS Converter  PhysicalDomain=network_engine_domain  SubClassName=ps_input  LeftPortType=input  RightPortType=output  PseudoPeriodic=off  Frequencies=[]  NoiseDistribution=none  NoiseParameters=[]  Unit=1  AffineConversion=off  FilteringAndDerivatives=zero  SimscapeFilterOrder=1  InputFilterTimeConstant=0.001  UdotUserProvided=1
  Simulink-PS Converter1 : nesl_utility/Simulink-PS Converter  PhysicalDomain=network_engine_domain  SubClassName=ps_input  LeftPortType=input  RightPortType=output  PseudoPeriodic=off  Frequencies=[]  NoiseDistribution=none  NoiseParameters=[]  Unit=1  AffineConversion=off  FilteringAndDerivatives=zero  SimscapeFilterOrder=1  InputFilterTimeConstant=.001  UdotUserProvided=[]
  Simulink-PS Converter2 : nesl_utility/Simulink-PS Converter  PhysicalDomain=network_engine_domain  SubClassName=ps_input  LeftPortType=input  RightPortType=output  PseudoPeriodic=off  Frequencies=[]  NoiseDistribution=none  NoiseParameters=[]  Unit=1  AffineConversion=off  FilteringAndDerivatives=zero  SimscapeFilterOrder=1  InputFilterTimeConstant=.001  UdotUserProvided=[]
  Sum : Sum  Inputs=|++
  To Workspace : ToWorkspace  VariableName=u_stance_hip_data  SampleTime=-1
  rad2deg : Gain  Gain=180/pi
  "rad2deg1 " : Gain  Gain=180/pi
  w : PMIOPort  Side=Right
  t : PMIOPort  Port=2  Side=Left
  q : PMIOPort  Port=3  Side=Right
  wires:
  PS-Simulink Converter1/1 -> "rad2deg1 "/1
  PS-Simulink Converter2/1 -> rad2deg/1
  rad2deg/1 -> Hip_S_lookup/1, Hip_D_lookup/1, Scope7/1, Product/2
  Hip_S_lookup/1 -> Product/1
  "rad2deg1 "/1 -> Product1/1, Scope6/1
  Product1/1 -> Sum/1, Scope2/1
  Product/1 -> Scope3/1, Sum/2
  Sum/1 -> Gain/1
  Gain/1 -> Simulink-PS Converter1/1, Scope1/1
  Hip_D_lookup/1 -> Product1/2
  Clock/1 -> Simulink-PS Converter2/1
  Stance_hip_moment/1 -> To Workspace/1, Simulink-PS Converter/1
  connections:
  w/RConn1 -- PS-Simulink Converter1/LConn1 -- Hard_Stop_Hip_L/LConn1
  Hard_Stop_Hip_L/RConn1 -- PS Add/LConn2
  Simulink-PS Converter1/RConn1 -- PS Add1/LConn2
  q/RConn1 -- PS-Simulink Converter2/LConn1
  PS Add1/RConn1 -- t/RConn1
  Simulink-PS Converter/RConn1 -- PS Add/LConn1
  Simulink-PS Converter2/RConn1 -- PS Lookup Table (1D)/LConn1
  PS Add/RConn1 -- PS Add2/LConn2
  PS Lookup Table (1D)/RConn1 -- PS Add2/LConn1
  PS Add2/RConn1 -- PS Add1/LConn1

== system ds1_plant/lag_hip_actuation/Stance_hip_PID ==
  Error : Inport
  Add : Sum  Inputs=+++
  Derivative : Derivative
  Gain : Gain  Gain=stance_hip_P
  Gain1 : Gain  Gain=stance_hip_I
  Gain2 : Gain  Gain=stance_hip_D
  Integrator : Integrator
  Saturation : Saturate  UpperLimit=100  LowerLimit=-100
  Scope : Scope
  Stance_hip_control_moment : Outport
  wires:
  Gain2/1 -> Add/3
  Gain1/1 -> Add/2
  Error/1 -> Derivative/1, Gain/1, Integrator/1
  Derivative/1 -> Gain2/1
  Gain/1 -> Add/1
  Integrator/1 -> Gain1/1
  Saturation/1 -> Stance_hip_control_moment/1
  Add/1 -> Scope/1, Saturation/1

== system ds1_plant/lag_knee_actuation/Hard_Stop_Knee_L ==
  Mechanical Rotational Reference : fl_lib/Mechanical/Rotational Elements/Mechanical Rotational Reference
  Rotational Simscape Intf (Library Block) : Subsystem
  Rotational Hard Stop : fl_lib/Mechanical/Rotational Elements/Rotational Hard Stop  upper_bnd=upper_bound rad  lower_bnd=lower_bound rad  stiff_up=contact_stiffness N*m/rad  stiff_low=contact_stiffness N*m/rad  D_up=contact_damping N*m/(rad/s)  D_low=contact_damping N*m/(rad/s)  model=3  transition=0.001 rad  w_specify=off  w_priority=None  w=0 rad/s  w_nominal_specify=off  w_nominal_unit=rad/s  w_nominal_value=1  t_specify=off  t_priority=None  t=0 N*m  t_nominal_specify=off  t_nominal_unit=N*m  t_nominal_value=1  phi_specify=on  phi_priority=High  phi=initial_angular_position rad  phi_nominal_specify=off  phi_nominal_unit=rad  phi_nominal_value=1
      settings: SourceProductName=Simscape  SourceProductBaseCode=SS
  T : PMIOPort  Side=Right
  w : PMIOPort  Port=2  Side=Left
  connections:
  Rotational Simscape Intf (Library Block)/RConn1 -- T/RConn1
  w/RConn1 -- Rotational Simscape Intf (Library Block)/LConn1
  Rotational Hard Stop/RConn1 -- Rotational Simscape Intf (Library Block)/RConn2
  Mechanical Rotational Reference/LConn1 -- Rotational Hard Stop/LConn1 -- Rotational Simscape Intf (Library Block)/LConn2

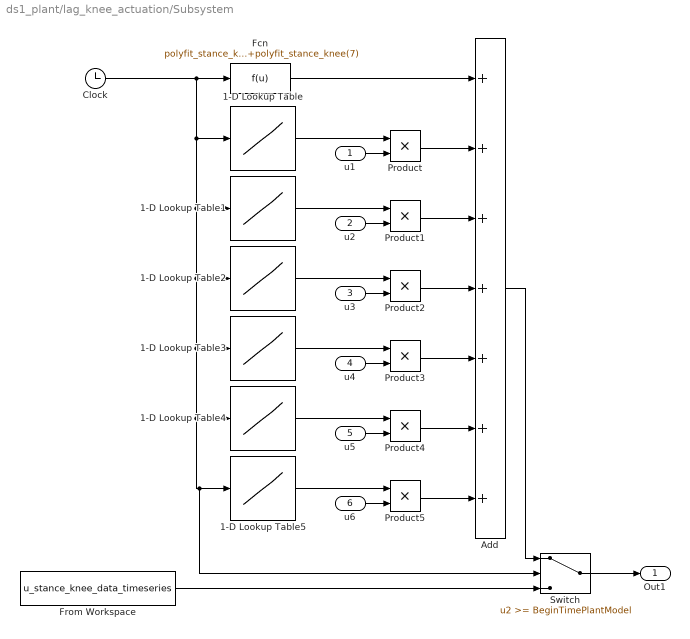
== system ds1_plant/lag_knee_actuation/Subsystem ==
  u1 : Inport
  u2 : Inport  Port=2
  u3 : Inport  Port=3
  u4 : Inport  Port=4
  u5 : Inport  Port=5
  u6 : Inport  Port=6
  1-D Lookup Table : Lookup_n-D  NumberOfTableDimensions=1  BreakpointsForDimension1=0:0.166/20:0.166  Table="[0.999949998749938\t0.00999949998749938\t9.99949998749938e-05\t9.99949998749938e-07\t9.99949998749938e-09\t9.99949998749938e-11\t9.99949998749938e-13\t9.99949998749938e-15\t9.99949998749938e-17\t9.99949998749938e-19\t9.99949998749938e-21\t9.99949998749938e-23\t9.99949998749938e-25\t9.99949998749938e-27\t9.99949998749938e-29\t9.99949998749938e-31\t9.99949998749938e-33\t9.99949998749938e-35\t9.99949998749938e-37\t9.99949998749938e-39\t9.99949998749938e-41]"  InternalRulePriority=Speed  RndMeth=Simplest  InputSameDT=on
  1-D Lookup Table1 : Lookup_n-D  NumberOfTableDimensions=1  BreakpointsForDimension1=0:0.166/20:0.166  Table="[-0.00999949998749938\t0.999750008750188\t0.0199960001250025\t0.000299945001625031\t3.99930002000038e-06\t4.99915002375044e-08\t5.99900002750050e-10\t6.99885003125056e-12\t7.99870003500063e-14\t8.99855003875069e-16\t9.99840004250075e-18\t1.09982500462508e-19\t1.19981000500009e-21\t1.29979500537509e-23\t1.39978000575010e-25\t1.49976500612511e-27\t1.59975000650011e-29\t1.69973500687512e-31\t1.79972000725013e-33\t1.89970500762513e-35\t1.99969000800014e-37]"  InternalRulePriority=Speed  RndMeth=Simplest  InputSameDT=on
  1-D Lookup Table2 : Lookup_n-D  NumberOfTableDimensions=1  BreakpointsForDimension1=0:0.166/20:0.166  Table="[9.99949998749938e-05\t-0.0199960001250025\t0.999350088747688\t0.0299865015624631\t0.000599770024249463\t9.99650034749263e-06\t1.49950504712403e-07\t2.09933506137377e-09\t2.79914007749848e-11\t3.59892009549815e-13\t4.49867511537279e-15\t5.49840513712241e-17\t6.59811016074699e-19\t7.79779018624654e-21\t9.09744521362106e-23\t1.04970752428705e-24\t1.19966802739950e-26\t1.35962603069944e-28\t1.52958153418688e-30\t1.70953453786182e-32\t1.89948504172425e-34]"  InternalRulePriority=Speed  RndMeth=Simplest  InputSameDT=on
  1-D Lookup Table3 : Lookup_n-D  NumberOfTableDimensions=1  BreakpointsForDimension1=0:0.166/20:0.166  Table="[-9.99949998749938e-07\t0.000299945001625031\t-0.0299865015624631\t0.998750358716438\t0.0399680074493850\t0.000999350133739838\t1.99885021798439e-05\t3.49814533160228e-07\t5.59720047896830e-09\t8.39598066445723e-11\t1.19944508924438e-12\t1.64925761673029e-14\t2.19903214934093e-16\t2.85876518751376e-18\t3.63845323168628e-20\t4.54809278229596e-22\t5.59768033978027e-24\t6.79721240457670e-26\t8.15668547712273e-28\t9.68609605785582e-30\t1.13954406472135e-31]"  InternalRulePriority=Speed  RndMeth=Simplest  InputSameDT=on
  1-D Lookup Table4 : Lookup_n-D  NumberOfTableDimensions=1  BreakpointsForDimension1=0:0.166/20:0.166  Table="[9.99949998749938e-09\t-3.99930002000038e-06\t0.000599770024249463\t-0.0399680074493850\t0.997950998567451\t0.0499375239337221\t0.00149852548805526\t3.49702589150649e-05\t6.99461150306087e-07\t1.25909723839627e-08\t2.09857536033307e-10\t3.29785552381578e-12\t4.94689323733114e-14\t7.14563951015331e-16\t1.00040408523439e-17\t1.36420392747520e-19\t1.81895722890139e-21\t2.37865729075538e-23\t3.05829696435827e-25\t3.87386865110997e-27\t4.84236430248908e-29]"  InternalRulePriority=Speed  RndMeth=Simplest  InputSameDT=on
  1-D Lookup Table5 : Lookup_n-D  NumberOfTableDimensions=1  BreakpointsForDimension1=0:0.166/20:0.166  Table="[-9.99949998749938e-11\t4.99915002375044e-08\t-9.99650034749263e-06\t0.000999350133739838\t-0.0499375239337221\t0.996952248088776\t0.0598920611597293\t0.00209709639706340\t5.59342282741959e-05\t1.25867752332421e-06\t2.51756490418445e-08\t4.61581047896514e-10\t7.91317131345719e-12\t1.28593499868373e-13\t2.00039890929054e-15\t3.00066657413218e-17\t4.36468860588449e-19\t6.18340796905681e-21\t8.56175943011575e-23\t1.16196690076089e-24\t1.54930534222886e-26]"  InternalRulePriority=Speed  RndMeth=Simplest  InputSameDT=on
  Add : Sum  Inputs=+++++++
  Clock : Clock
  Fcn : Fcn  Expr=polyfit_stance_knee(1)*u^6+polyfit_stance_knee(2)*u^5+polyfit_stance_knee(3)*u^4+polyfit_stance_knee(4)*u^3+polyfit_stance_knee(5)*u^2+polyfit_stance_knee(6)*u+polyfit_stance_knee(7)
  From Workspace : FromWorkspace  VariableName=u_stance_knee_data_timeseries  SampleTime=0
  Product{,1..5} (6 alike) : Product
  Switch : Switch  Threshold=BeginTimePlantModel
  Out1 : Outport
  wires:
  Clock/1 -> 1-D Lookup Table/1, 1-D Lookup Table1/1, 1-D Lookup Table2/1, 1-D Lookup Table3/1, 1-D Lookup Table4/1, 1-D Lookup Table5/1, Switch/2, Fcn/1
  1-D Lookup Table/1 -> Product/1
  u1/1 -> Product/2
  1-D Lookup Table1/1 -> Product1/1
  u2/1 -> Product1/2
  1-D Lookup Table2/1 -> Product2/1
  u3/1 -> Product2/2
  1-D Lookup Table3/1 -> Product3/1
  u4/1 -> Product3/2
  1-D Lookup Table4/1 -> Product4/1
  u5/1 -> Product4/2
  1-D Lookup Table5/1 -> Product5/1
  u6/1 -> Product5/2
  Fcn/1 -> Add/1
  Product/1 -> Add/2
  Product1/1 -> Add/3
  Product2/1 -> Add/4
  Product3/1 -> Add/5
  Product4/1 -> Add/6
  Product5/1 -> Add/7
  Switch/1 -> Out1/1
  Add/1 -> Switch/1
  From Workspace/1 -> Switch/3

== system ds1_plant/lead foot/Heel_GRF ==
  External Force  and Torque : sm_lib/Forces and Torques/External Force and Torque  ForceResolutionFrame=World  EnableForceX=off  EnableForceY=on  EnableForceZ=on  EnableForce=off  TorqueResolutionFrame=AttachedFrame  EnableTorqueX=off  EnableTorqueY=off  EnableTorqueZ=off  EnableTorque=off
  Heel Sensor : sm_lib/Frames and Transforms/Transform Sensor  MeasurementFrame=World  SenseAngle=off  SenseAxis=off  SenseAngle1=off  SenseAngle2=off  SenseAngle3=off  SenseQ=off  SenseR=off  SenseOmegaX=off  SenseOmegaY=off  SenseOmegaZ=off  SenseOmega1=off  SenseOmega2=off  SenseOmega3=off  SenseQDot=off  SenseRDot=off  SenseAlphaX=off  SenseAlphaY=off  SenseAlphaZ=off  SenseAlpha1=off  SenseAlpha2=off  SenseAlpha3=off  SenseQDDot=off  SenseRDDot=off  SenseX=off  SenseY=on  SenseZ=on  SenseRad=off  SenseAzim=off  SenseDist=off  SenseInc=off  SenseXDot=off  SenseYDot=on  SenseZDot=on  SenseRadDot=off  SenseAzimDot=off  SenseDistDot=off  SenseIncDot=off  SenseXDDot=off  SenseYDDot=off  SenseZDDot=off  SenseRadDDot=off  SenseAzimDDot=off  SenseDistDDot=off  SenseIncDDot=off
  Subsystem : Subsystem
  Subsystem1 : Subsystem
  Heel : PMIOPort  Side=Left
  connections:
  Subsystem1/RConn1 -- External Force  and Torque/LConn1
  External Force  and Torque/LConn2 -- Subsystem/RConn1
  Heel Sensor/RConn4 -- Subsystem1/LConn3
  Heel Sensor/RConn2 -- Subsystem1/LConn2
  Heel Sensor/RConn5 -- Subsystem/LConn2
  Heel/RConn1 -- Heel Sensor/RConn1 -- External Force  and Torque/RConn1
  Subsystem/LConn1 -- Subsystem1/LConn1 -- Heel Sensor/RConn3

== system ds1_plant/lead foot/Toe_GRF  ==
  External Force  and Torque : sm_lib/Forces and Torques/External Force and Torque  ForceResolutionFrame=World  EnableForceX=off  EnableForceY=on  EnableForceZ=on  EnableForce=off  TorqueResolutionFrame=AttachedFrame  EnableTorqueX=off  EnableTorqueY=off  EnableTorqueZ=off  EnableTorque=off
  Subsystem : Subsystem
  Subsystem1 : Subsystem
  Toe Sensor : sm_lib/Frames and Transforms/Transform Sensor  MeasurementFrame=World  SenseAngle=off  SenseAxis=off  SenseAngle1=off  SenseAngle2=off  SenseAngle3=off  SenseQ=off  SenseR=off  SenseOmegaX=off  SenseOmegaY=off  SenseOmegaZ=off  SenseOmega1=off  SenseOmega2=off  SenseOmega3=off  SenseQDot=off  SenseRDot=off  SenseAlphaX=off  SenseAlphaY=off  SenseAlphaZ=off  SenseAlpha1=off  SenseAlpha2=off  SenseAlpha3=off  SenseQDDot=off  SenseRDDot=off  SenseX=off  SenseY=on  SenseZ=on  SenseRad=off  SenseAzim=off  SenseDist=off  SenseInc=off  SenseXDot=off  SenseYDot=on  SenseZDot=on  SenseRadDot=off  SenseAzimDot=off  SenseDistDot=off  SenseIncDot=off  SenseXDDot=off  SenseYDDot=off  SenseZDDot=off  SenseRadDDot=off  SenseAzimDDot=off  SenseDistDDot=off  SenseIncDDot=off
  Toe : PMIOPort  Side=Left
  connections:
  External Force  and Torque/LConn1 -- Subsystem1/RConn1
  Subsystem/RConn1 -- External Force  and Torque/LConn2
  Toe Sensor/RConn4 -- Subsystem1/LConn3
  Toe Sensor/RConn2 -- Subsystem1/LConn2
  Toe Sensor/RConn5 -- Subsystem/LConn2
  Toe/RConn1 -- Toe Sensor/RConn1 -- External Force  and Torque/RConn1
  Subsystem/LConn1 -- Subsystem1/LConn1 -- Toe Sensor/RConn3

== system ds1_plant/lead_ankle_actuation/Hard_Stop_Ankle_L1 ==
  Mechanical Rotational Reference : fl_lib/Mechanical/Rotational Elements/Mechanical Rotational Reference
  Rotational Simscape Intf (Library Block) : Subsystem
  Rotational Hard Stop : fl_lib/Mechanical/Rotational Elements/Rotational Hard Stop  upper_bnd=upper_bound rad  lower_bnd=lower_bound rad  stiff_up=contact_stiffness N*m/rad  stiff_low=contact_stiffness N*m/rad  D_up=contact_damping N*m/(rad/s)  D_low=contact_damping N*m/(rad/s)  model=3  transition=0.001 rad  w_specify=off  w_priority=None  w=0 rad/s  w_nominal_specify=off  w_nominal_unit=rad/s  w_nominal_value=1  t_specify=off  t_priority=None  t=0 N*m  t_nominal_specify=off  t_nominal_unit=N*m  t_nominal_value=1  phi_specify=on  phi_priority=High  phi=initial_angular_position rad  phi_nominal_specify=off  phi_nominal_unit=rad  phi_nominal_value=1
      settings: SourceProductName=Simscape  SourceProductBaseCode=SS
  T : PMIOPort  Side=Right
  w : PMIOPort  Port=2  Side=Left
  connections:
  Rotational Simscape Intf (Library Block)/LConn2 -- Rotational Hard Stop/LConn1 -- Mechanical Rotational Reference/LConn1
  Rotational Hard Stop/RConn1 -- Rotational Simscape Intf (Library Block)/RConn2
  w/RConn1 -- Rotational Simscape Intf (Library Block)/LConn1
  Rotational Simscape Intf (Library Block)/RConn1 -- T/RConn1
